simulink model "sampleModel16"  (R2021b)
settings: Solver=VariableStepAuto  StartTime=0.0  StopTime=10.0  RelTol=1e-3
undefined symbols (not defined in the file or in its folder): Newton, Raphson
libraries: simulink x6
settings Model: Creator=user  LastModifiedBy=user

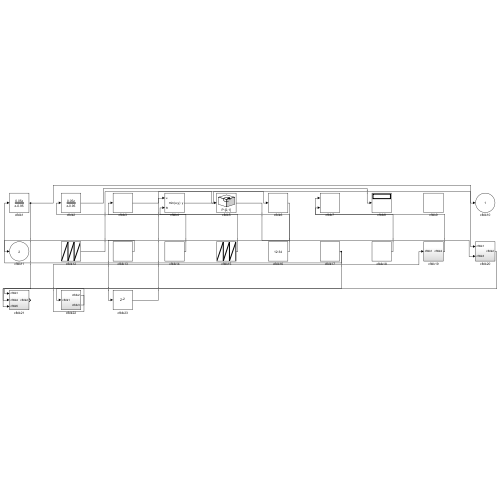
[thumbnail: Simulink's stored preview of the top-level diagram]
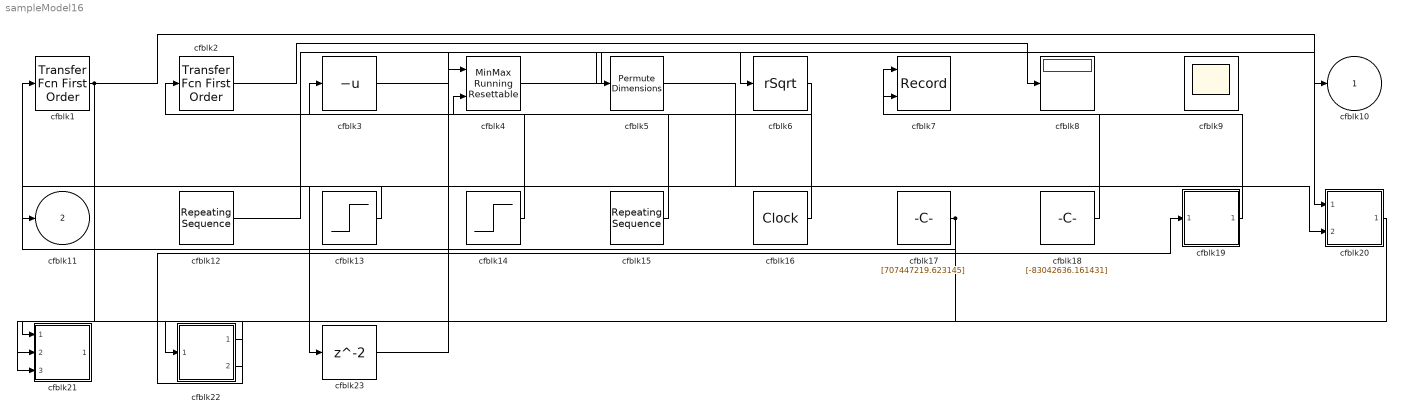
== system sampleModel16 ==
  cfblk1 : simulink/Discrete/Transfer Fcn First Order  PoleZ=0.95  ICPrevOutput=0.0  DoSatur=off
  cfblk12 : simulink/Sources/Repeating Sequence  rep_seq_t=[0 2]  rep_seq_y=[90868516.516904, 498567434.662939]
  cfblk13 : Step  Time=[7.000000]  Before=[-93530363.756993]  After=[-850501123.088467]  SampleTime=0
  cfblk14 : Step  Time=[33.000000]  Before=[407303283.856135]  After=[837901136.616507]  SampleTime=0
  cfblk15 : simulink/Sources/Repeating Sequence  rep_seq_t=[0 2]  rep_seq_y=[320143816.801906, 380209838.563271]
  cfblk16 : DigitalClock
  cfblk17 : Constant  Value=[707447219.623145]  SampleTime=1
  cfblk18 : Constant  Value=[-83042636.161431]  SampleTime=1
  cfblk19 : Subsystem
  cfblk2 : simulink/Discrete/Transfer Fcn First Order  PoleZ=0.95  ICPrevOutput=0.0  DoSatur=off
  cfblk20 : Subsystem
  cfblk21 : Subsystem
  cfblk22 : Subsystem
  cfblk23 : Delay  SampleTime=1
  cfblk3 : UnaryMinus
  cfblk4 : simulink/Math Operations/MinMax Running Resettable  Function=min  vinit=0.0
  cfblk5 : PermuteDimensions
  cfblk6 : Sqrt  Operator=rSqrt  AlgorithmType=Newton-Raphson  SaturateOnIntegerOverflow=on
  cfblk7 : Record  FileSettingsInternal="{\"entries\":[{\"content\":{\"excelSettings\":{\"content\":{},\"type\":\"Streamout.ExcelSettings\"}},\"type\":\"Streamout.FileSettingStorage\",\"uuid\":\"dcc2fbcf-9eeb-4f5c-ab26-c068f2b21078\"}],\"packageUris\":[\"http://schema.mathworks.com/mf0/streamout_blocks/R2020a\"],\"version\":\"1.0\"}"  Layout=[1 1]  SignalsInternal="{\"entries\":[{\"content\":{\"signals\":[{\"content\":{\"blockPath\":[\"sampleModel16/cfblk7\"],\"channel\":[],\"dimensions\":[1],\"domain\":\"sampleModel16/cfblk7\",\"lineColor\":\"#a2142f\",\"plots\":[1],\"port\":1,\"sid\":[\"\"],\"signalID\":642,\"signalName\":\"cfblk18\"},\"type\":\"RecordBlkView.Signal\",\"uuid\":\"e116d46d-13e1-49b0-9399-3440b7c1db51\"},{\"content\":{\"blockPath\":[\"sampleModel16/cfblk7\"],\"channel\":[],\"dimensions\":[1,1],\"domain\":\"sampleModel16/cfblk7\",\"lineColor\":\"#139fff\",\"plots\":[1],\"port\":2,\"sid\":[\"\"],\"signalID\":646,\"signalName\":\"cfblk19\"},\"type\":\"RecordBlkView.Signal\",\"uuid\":\"f0d7a045-2ead-4924-ac95-26a522785816\"}]},\"type\":\"RecordBlkView.InputSignals\",\"uuid\":\"afbacf41-43d7-4eae-9335-c9f4eb6fbf70\"}],\"packageUris\":[\"http://schema.mathworks.com/mf0/streamout_blocks/R2020a\"],\"version\":\"1.0\"}"  VisualizationBindings="{\"xyplotplugin\":{\"info\":[{\"series\":[{\"bindingParametersList\":[{\"parameter\":\"X-Axis\",\"signalID\":642,\"signalName\":\"cfblk18\"},{\"parameter\":\"Y-Axis\",\"signalID\":646,\"signalName\":\"cfblk19\"}],\"seriesID\":42967}],\"subplotID\":1}]}}"  CompatibilityTag=XY
  cfblk8 : Display
  cfblk9 : Scope
      settings: Floating=on
  cfblk10 : Outport
  cfblk11 : Outport  Port=2
  wires:
  cfblk4/1 -> cfblk6/1
  cfblk16/1 -> cfblk3/1
  cfblk12/1 -> cfblk5/1
  cfblk17/1 -> cfblk1/1, cfblk21/2(cfblk4)
  cfblk20/1(cfblk2) -> cfblk22/1(cfblk1)
  cfblk15/1 -> cfblk2/1
  cfblk2/1 -> cfblk8/1
  cfblk13/1 -> cfblk11/1
  cfblk22/1(cfblk2) -> cfblk19/1(cfblk1)
  cfblk14/1 -> cfblk4/2
  cfblk1/1 -> cfblk20/1(cfblk1), cfblk21/3(cfblk5)
  cfblk5/1 -> cfblk20/2(cfblk3)
  cfblk3/1 -> cfblk10/1
  cfblk18/1 -> cfblk7/1
  cfblk19/1(cfblk2) -> cfblk7/2
  cfblk22/2(cfblk3) -> cfblk21/1(cfblk1)
  cfblk6/1 -> cfblk23/1
  cfblk23/1 -> cfblk4/1

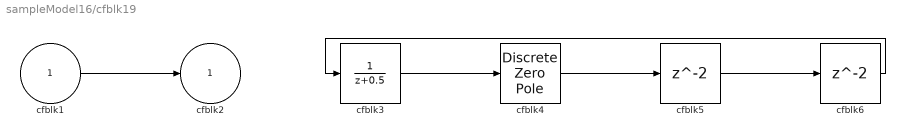
== system sampleModel16/cfblk19 ==
  cfblk1 : Inport
  cfblk3 : DiscreteTransferFcn  SampleTime=1
  cfblk4 : DiscreteZeroPole  Poles=[0 0.5]  Gain=1
  cfblk5 : Delay  SampleTime=1
  cfblk6 : Delay  SampleTime=1
  cfblk2 : Outport
  wires:
  cfblk1/1 -> cfblk2/1
  cfblk3/1 -> cfblk4/1
  cfblk4/1 -> cfblk5/1
  cfblk5/1 -> cfblk6/1
  cfblk6/1 -> cfblk3/1

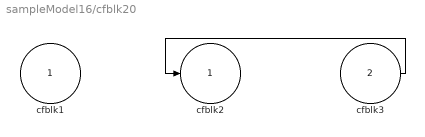
== system sampleModel16/cfblk20 ==
  cfblk1 : Inport
  cfblk3 : Inport  Port=2
  cfblk2 : Outport
  wires:
  cfblk3/1 -> cfblk2/1

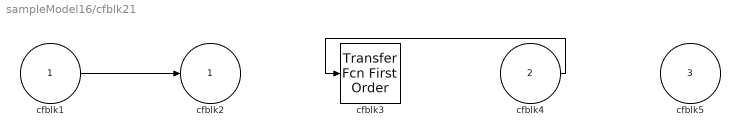
== system sampleModel16/cfblk21 ==
  cfblk1 : Inport
  cfblk4 : Inport  Port=2
  cfblk5 : Inport  Port=3
  cfblk3 : simulink/Discrete/Transfer Fcn First Order  PoleZ=0.95  ICPrevOutput=0.0  DoSatur=off
  cfblk2 : Outport
  wires:
  cfblk1/1 -> cfblk2/1
  cfblk4/1 -> cfblk3/1

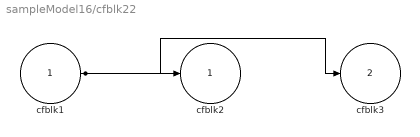
== system sampleModel16/cfblk22 ==
  cfblk1 : Inport
  cfblk2 : Outport
  cfblk3 : Outport  Port=2
  wires:
  cfblk1/1 -> cfblk2/1, cfblk3/1
